simulink model "demoDINA_PCSSP"  (Simulink 8.0)
settings: Solver=ode1  SolverMode=SingleTasking  StartTime=0.0  StopTime=100.1  FixedStep=SimStep  RelTol=1e-3
InitFcn:
  | init_param_PCS6;
values from neighbouring files (symbols this model uses):
  n_gaps = 6    [init_param_PCS6.m]
  ncam = 100    [init_param_PCS6.m]
  npf = 15    [init_param_PCS6.m]
  SimStep = 2e-3    (= 0.002)    [init_param_PCS6.m]
  Time_stop = 1530    [init_param_PCS6.m]
undefined symbols (not defined in the file or in its folder): c_eob, dt_end_sim, dtpl_term_l, elong_ref, g1_ref, g1_ref_term, g2_ref, g2_ref_term, g3_ref, g3_ref_term, g4_ref, g4_ref_term, g5_ref, g5_ref_term, g6_ref, g6_ref_term, Ics1_eob, Ip_0, Ip_div, k_gaplim, n_mc, Ratemc_low, Ratemc_up, ref_ramp, scr_data, scr_PF, t_eob2, t_tran2D, Tfmc, Vmc_low, Vmc_up, VS_low, VS_up
libraries: simulink x5
settings Model: Creator=invite  LastModifiedBy=medveds  ExtModeAutoUpdateStatusClock=off  TunableVars=K,num  TunableVarsStorageClass=Auto,Auto  TunableVarsTypeQualifier=,  BufferReuse=off
settings DataIOCC: SignalLoggingSaveFormat=ModelDataLogs
settings OptimizationCC: BlockReduction=off  BooleanDataType=off  ConditionallyExecuteInputs=off  OptimizeBlockIOStorage=off  BufferReuse=off  ExpressionFolding=off  LocalBlockOutputs=off  InitFltsAndDblsToZero=on  AccelVerboseBuild=on
settings DebuggingCC: FcnCallInpInsideContextMsg=UseLocalSettings  SFcnCompatibilityMsg=warning  StrictBusMsg=Warning
settings SFSimCC: SimParseCustomCode=off  SimBuildMode=sf_make
settings CodeAppCC: CustomSymbolStrType=$N$R$M_T
settings GRTTargetCC: CombineOutputUpdateFcns=off  GRTInterface=on

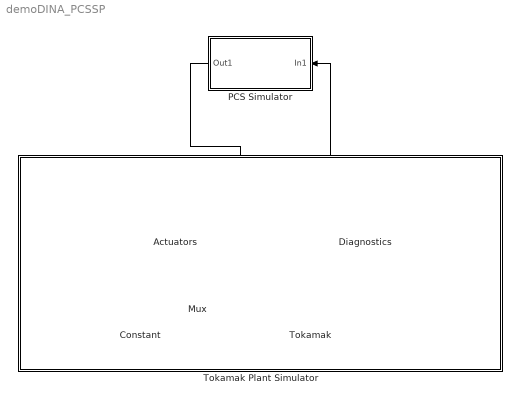
== system demoDINA_PCSSP ==
  Actuators : Subsystem
  Constant : Constant  Value=5  SampleTime=-1
  Diagnostics : Subsystem
  Mux : Mux  Inputs=2
  PCS Simulator : Subsystem
  Tokamak : S-Function  FunctionName=simimasdialogPCSSP  EnableBusSupport=off
  Tokamak Plant Simulator : Subsystem
      mask Display: disp(' ')
  wires:
  Mux/1 -> Tokamak/1
  Constant/1 -> Mux/2
  PCS Simulator/1(Out1) -> Actuators/1(In1)
  Actuators/1(Out1) -> Mux/1
  Tokamak/1 -> Diagnostics/1(In1)
  Diagnostics/1(Out1) -> PCS Simulator/1(In1)

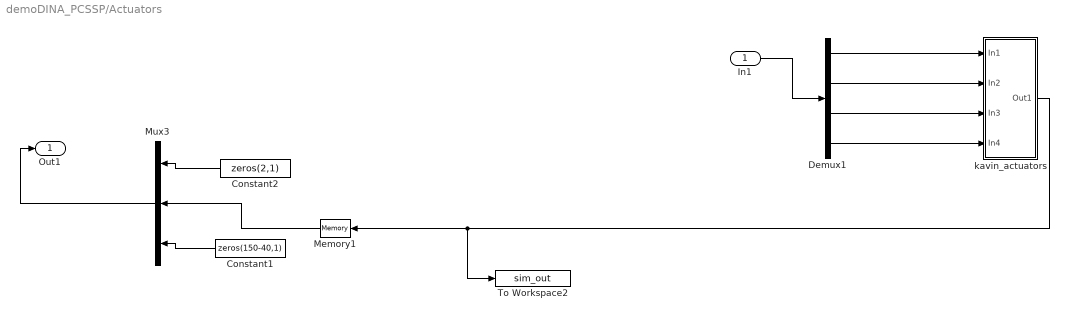
== system demoDINA_PCSSP/Actuators ==
  In1 : Inport
  Constant1 : Constant  Value=zeros(150-40,1)
  Constant2 : Constant  Value=zeros(2,1)
  Demux1 : Demux  Outputs=[n_mc 1 n_mc 12]
  Memory1 : Memory
  Mux3 : Mux  Inputs=3
  To Workspace2 : ToWorkspace  VariableName=sim_out
  kavin_actuators : Subsystem
  Out1 : Outport
  wires:
  In1/1 -> Demux1/1
  Mux3/1 -> Out1/1
  kavin_actuators/1(Out1) -> To Workspace2/1, Memory1/1
  Demux1/1 -> kavin_actuators/1(In1)
  Demux1/2 -> kavin_actuators/2(In2)
  Demux1/3 -> kavin_actuators/3(In3)
  Demux1/4 -> kavin_actuators/4(In4)
  Constant1/1 -> Mux3/3
  Memory1/1 -> Mux3/2
  Constant2/1 -> Mux3/1

== system demoDINA_PCSSP/Diagnostics ==
  In1 : Inport
  Out1 : Outport
  wires:
  In1/1 -> Out1/1

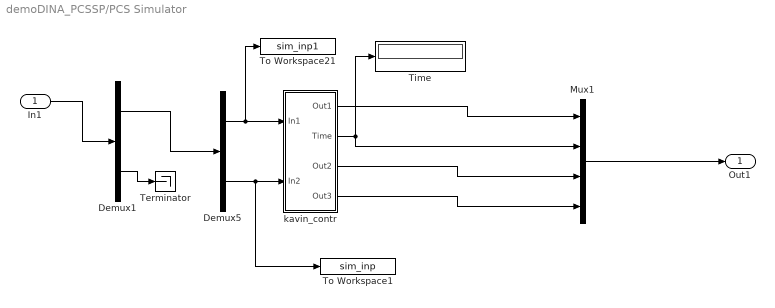
== system demoDINA_PCSSP/PCS Simulator ==
  In1 : Inport
  Demux1 : Demux  Outputs=[138 12]
  Demux5 : Demux  Outputs=[15 123]
  Mux1 : Mux
  Terminator : Terminator
  Time : Display
  To Workspace1 : ToWorkspace  VariableName=sim_inp
  To Workspace21 : ToWorkspace  VariableName=sim_inp1
  kavin_contr : Subsystem
  Out1 : Outport
  wires:
  Demux5/1 -> kavin_contr/1(In1), To Workspace21/1
  Demux5/2 -> kavin_contr/2(In2), To Workspace1/1
  Demux1/1 -> Demux5/1
  In1/1 -> Demux1/1
  Demux1/2 -> Terminator/1
  kavin_contr/2(Time) -> Mux1/2, Time/1
  kavin_contr/1(Out1) -> Mux1/1
  kavin_contr/3(Out2) -> Mux1/3
  kavin_contr/4(Out3) -> Mux1/4
  Mux1/1 -> Out1/1

== system demoDINA_PCSSP/Tokamak Plant Simulator ==

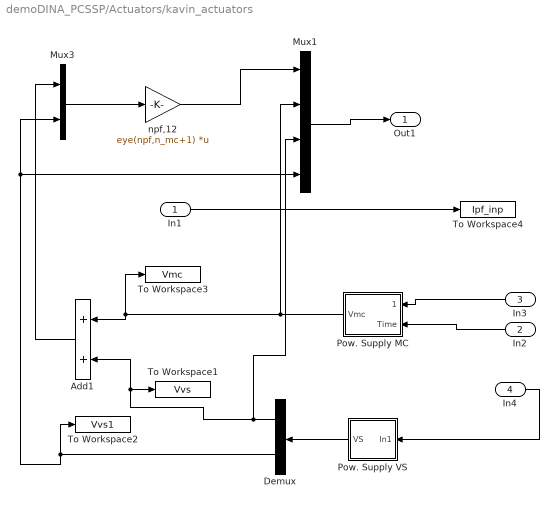
== system demoDINA_PCSSP/Actuators/kavin_actuators ==
  In1 : Inport
  In2 : Inport  Port=2
  In3 : Inport  Port=3
  In4 : Inport  Port=4
  Add1 : Sum
  Demux : Demux  Outputs=[n_mc 1]
  Mux1 : Mux
  Mux3 : Mux  Inputs=2
  "Pow. Supply MC " : Subsystem
  Pow. Supply VS : Subsystem
  To Workspace1 : ToWorkspace  VariableName=Vvs
  To Workspace2 : ToWorkspace  VariableName=Vvs1
  To Workspace3 : ToWorkspace  VariableName=Vmc
  To Workspace4 : ToWorkspace  VariableName=Ipf_inp
  npf,12 : Gain  Gain=eye(npf,n_mc+1)  Multiplication=Matrix(K*u)
  Out1 : Outport
  wires:
  Add1/1 -> Mux3/1
  Mux3/1 -> npf,12/1
  Demux/2 -> Mux1/4, Mux3/2, To Workspace2/1
  Demux/1 -> Mux1/3, To Workspace1/1, Add1/2
  In4/1 -> Pow. Supply VS/1(In1)
  Pow. Supply VS/1(VS) -> Demux/1
  In3/1 -> "Pow. Supply MC "/1(Vcontr)
  In2/1 -> "Pow. Supply MC "/2(Time)
  In1/1 -> To Workspace4/1
  npf,12/1 -> Mux1/1
  "Pow. Supply MC "/1(Vmc) -> Add1/1, To Workspace3/1, Mux1/2
  Mux1/1 -> Out1/1

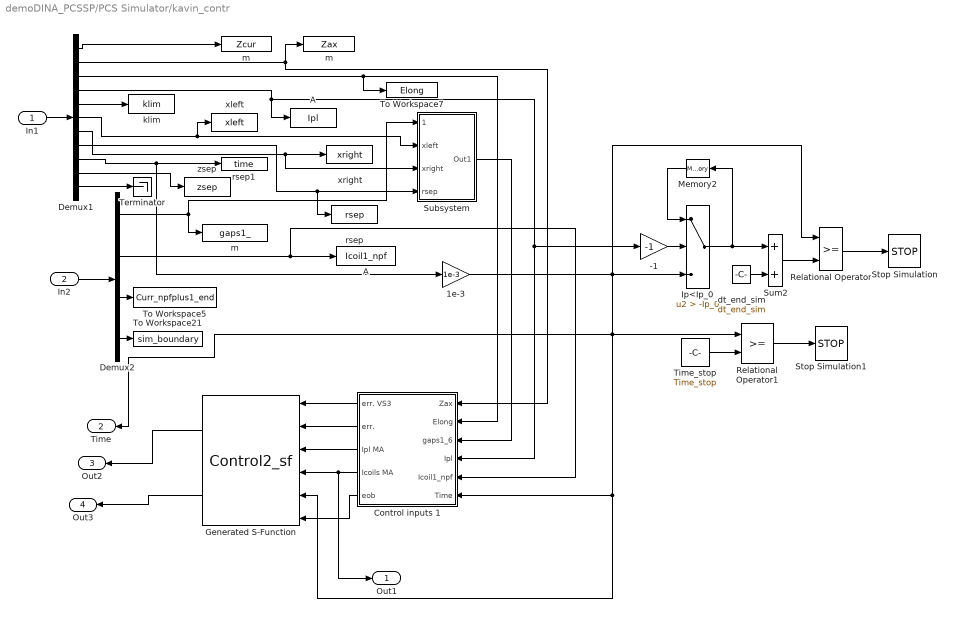
== system demoDINA_PCSSP/PCS Simulator/kavin_contr ==
  In1 : Inport
  In2 : Inport  Port=2
  -1 : Gain  Gain=-1
  1e-3 : Gain  Gain=1e-3
  A : ToWorkspace  VariableName=Ipl
  "A  " : ToWorkspace  VariableName=Icoil1_npf
  Control inputs 1 : Subsystem
  Demux1 : Demux  Outputs=[1 1 1 1 1 1 1 1 1 1 5 ]
  Demux2 : Demux  Outputs=[n_gaps npf ncam 2]
  Generated S-Function : S-Function  FunctionName=Control2_sf  SFunctionModules=""  EnableBusSupport=off  mask{rtw_sf_name=Control2_sf, showVar=off}
      mask prompts: rtw_sf_name "Simulink:masks:GenSFuncName_MP"; showVar "Simulink:masks:GenSFuncShowModuleList_MP"
      mask help: Simulink:masks:GenSFuncDesc_MD
      mask init:
      | displist = '';
      | if ~strcmp(get_param(gcb, 'FunctionName'), rtw_sf_name);
      |   set_param(gcb, 'FunctionName', rtw_sf_name);
      | end
      | % Check if we are generating code
      | rtw_mode = false;
      | if strcmpi(get_param(bdroot(gcb),'SimulationStatus'),'Initializing')
      | 	rtw_mode = strcmpi(get_param(bdroot(gcb),'BuildingRTWCode'),'on') && ...
      | 		~strcmpi(get_param(bdroot(gcb),'TargetStyle'),'SimulationTarget');
      | end
      | if showVar || rtw_mode
      | 	if exist('rtwsfunc') == 2 | exist('rtwsfunc') == 6
      | 		tmplist = rtwsfunc(rtw_sf_name,gcb);
      | 		tmplist = DAStudio.message('Simulink:masks:GenSFuncListOfModules_IC', tmplist);
      | 	elseif showVar
      | 		tmplist1 = DAStudio.message('Simulink:masks:GenSFuncListOfModules_IC', '');
      |         tmplist2 = DAStudio.message('Simulink:masks:GenSFuncNotLicensed_IC');
      |         tmplist = [tmplist1 tmplist2];
      |  	end
      | end
      | if showVar
      |   displist = tmplist;
      | end
      settings: CopyFcn=|
      | if ~strcmp(get_param(gcb,'Linkstatus'),'none') && ...
      | ~strcmp(get_param(gcb,'Linkstatus'),'implicit')
      |   set_param(gcb,'LinkStatus','none');
      | end
      mask Help: eval('feval(''rtwprivate'',''rtwhelpview'',''rtw_sfcn_block'')');
      mask Display:
      | port_label('input',1,'err. VS3');
      | port_label('input',2,'err.');
      | port_label('input',3,'Ipl MA');
      | port_label('input',4,'Icoils MA');
      | port_label('input',5,'Time');
      | port_label('input',6,'eob');
      | port_label('output',1,'Vmc control');
      | port_label('output',2,'Vvs control');
  "Ip<Ip_0 " : Switch  Criteria=u2 > Threshold  Threshold=-Ip_0
  Memory2 : Memory
  Relational Operator : RelationalOperator  OutDataTypeStr=boolean
  Relational Operator1 : RelationalOperator  OutDataTypeStr=boolean
  Stop Simulation : Stop
  Stop Simulation1 : Stop
  Subsystem : Subsystem
  Sum2 : Sum
  Terminator : Terminator
  Time_stop : Constant  Value=Time_stop
  To Workspace21 : ToWorkspace  VariableName=sim_boundary
      settings: Decimation=DecimShape
  To Workspace5 : ToWorkspace  VariableName=Curr_npfplus1_end
  To Workspace7 : ToWorkspace  VariableName=Elong
  dt_end_sim : Constant  Value=dt_end_sim
  klim : ToWorkspace  VariableName=klim
  m : ToWorkspace  VariableName=gaps1_
  "m  " : ToWorkspace  VariableName=Zax
  "m   " : ToWorkspace  VariableName=Zcur
  rsep : ToWorkspace  VariableName=rsep
  rsep1 : ToWorkspace  VariableName=time
  xleft : ToWorkspace  VariableName=xleft
  xright : ToWorkspace  VariableName=xright
  zsep : ToWorkspace  VariableName=zsep
  Out1 : Outport
  Time : Outport  Port=2
  Out2 : Outport  Port=3
  Out3 : Outport  Port=4
  wires:
  Demux1/2 -> "m  "/1, Control inputs 1/1(Zax)
  Demux1/1 -> "m   "/1
  Demux1/3 -> To Workspace7/1, Control inputs 1/2(Elong)
  Demux2/4 -> To Workspace21/1
  Demux1/4 -> A/1, Control inputs 1/4(Ipl), -1/1
  Demux2/3 -> To Workspace5/1
  Demux2/2 -> "A  "/1, Control inputs 1/5(Icoil1_npf)
  Control inputs 1/1(err. VS3) -> Generated S-Function/1
  Control inputs 1/2(err.) -> Generated S-Function/2
  Control inputs 1/3(Ipl MA) -> Generated S-Function/3
  Control inputs 1/4(Icoils MA) -> Out1/1, Generated S-Function/4
  In1/1 -> Demux1/1
  In2/1 -> Demux2/1
  Demux1/5 -> klim/1
  Demux1/6 -> xleft/1, Subsystem/2(xleft)
  Demux1/7 -> xright/1, Subsystem/3(xright)
  Demux1/8 -> rsep/1, Subsystem/4(rsep)
  Demux2/1 -> m/1, Subsystem/1(gaps1_6)
  Subsystem/1(Out1) -> Control inputs 1/3(gaps1_6)
  Demux1/11 -> Terminator/1
  Demux1/9 -> rsep1/1, 1e-3/1
  Demux1/10 -> zsep/1
  1e-3/1 -> "Ip<Ip_0 "/3, Relational Operator/1, Time/1, Generated S-Function/5, Control inputs 1/6(Time), Relational Operator1/1
  Relational Operator/1 -> Stop Simulation/1
  -1/1 -> "Ip<Ip_0 "/2
  "Ip<Ip_0 "/1 -> Memory2/1, Sum2/1
  Memory2/1 -> "Ip<Ip_0 "/1
  Sum2/1 -> Relational Operator/2
  dt_end_sim/1 -> Sum2/2
  Relational Operator1/1 -> Stop Simulation1/1
  Time_stop/1 -> Relational Operator1/2
  Control inputs 1/5(eob) -> Generated S-Function/6
  Generated S-Function/1 -> Out2/1
  Generated S-Function/2 -> Out3/1

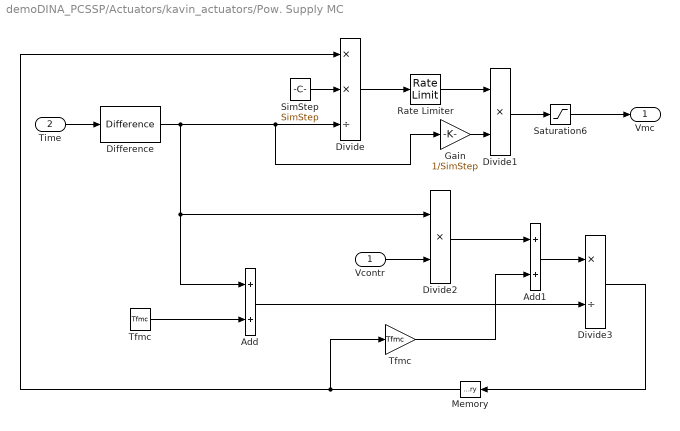
== system demoDINA_PCSSP/Actuators/kavin_actuators/Pow. Supply MC  ==
  Vcontr : Inport
  Time : Inport  Port=2
  Add : Sum
  Add1 : Sum
  Difference : simulink/Discrete/Difference  ICPrevInput=0.0  InputProcessing=Inherited  OutMin=[]  OutMax=[]  OutDataType=sfix(16)  OutScaling=2^-10  DoSatur=off
  Divide : Product  Inputs=**/
  Divide1 : Product  Inputs=**
  Divide2 : Product  Inputs=**
  Divide3 : Product  Inputs=*/
  Gain : Gain  Gain=1/SimStep
  Memory : Memory
  Rate Limiter : RateLimiter  RisingSlewLimit=Ratemc_up  FallingSlewLimit=Ratemc_low  SampleTimeMode=inherited
  Saturation6 : Saturate  UpperLimit=Vmc_up  LowerLimit=Vmc_low
  SimStep : Constant  Value=SimStep
  Tfmc : Constant  Value=Tfmc
  "Tfmc " : Gain  Gain=Tfmc
  Vmc : Outport
  wires:
  Saturation6/1 -> Vmc/1
  Time/1 -> Difference/1
  SimStep/1 -> Divide/2
  Difference/1 -> Divide/3, Gain/1, Divide2/1, Add/1
  Divide/1 -> Rate Limiter/1
  Rate Limiter/1 -> Divide1/1
  Divide1/1 -> Saturation6/1
  Gain/1 -> Divide1/2
  Tfmc/1 -> Add/2
  Divide2/1 -> Add1/1
  Memory/1 -> Divide/1, "Tfmc "/1
  Vcontr/1 -> Divide2/2
  "Tfmc "/1 -> Add1/2
  Add1/1 -> Divide3/1
  Divide3/1 -> Memory/1
  Add/1 -> Divide3/2

== system demoDINA_PCSSP/Actuators/kavin_actuators/Pow. Supply VS ==
  In1 : Inport
  Saturation VS : Saturate  UpperLimit=VS_up  LowerLimit=VS_low
  VS : Outport
  wires:
  In1/1 -> Saturation VS/1
  Saturation VS/1 -> VS/1

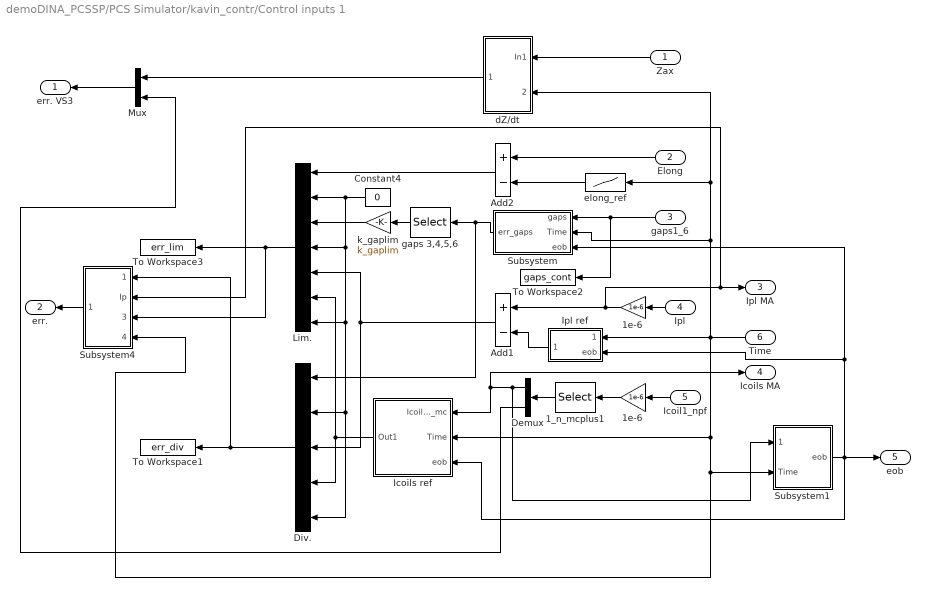
== system demoDINA_PCSSP/PCS Simulator/kavin_contr/Control inputs 1 ==
  Zax : Inport
  Elong : Inport  Port=2
  gaps1_6 : Inport  Port=3
  Ipl : Inport  Port=4
  Icoil1_npf : Inport  Port=5
  Time : Inport  Port=6
  1_n_mcplus1 : Selector  InputPortWidth=npf  IndexOptions=Index vector (dialog)  Indices=[1:n_mc+1]  OutputSizes=1
  1e-6 : Gain  Gain=1e-6
  "1e-6   " : Gain  Gain=1e-6
  Add1 : Sum  Inputs=+-
  Add2 : Sum  Inputs=+-
  Constant4 : Constant  Value=0  VectorParams1D=off
  Demux : Demux  Outputs=[n_mc 1]
  "Div. " : Mux  Inputs=5
  Icoils ref : Subsystem
  Ipl ref : Subsystem
  "Lim. " : Mux  Inputs=7
  Mux : Mux  Inputs=2
  Subsystem : Subsystem
  Subsystem1 : Subsystem
  Subsystem4 : Subsystem
  To Workspace1 : ToWorkspace  VariableName=err_div
  To Workspace2 : ToWorkspace  VariableName=gaps_cont
  To Workspace3 : ToWorkspace  VariableName=err_lim
  dZ/dt : Subsystem
  elong_ref : Lookup  InputValues=elong_ref(:,1)  Table=elong_ref(:,2)
  gaps 3,4,5,6 : Selector  InputPortWidth=6  IndexOptions=Index vector (dialog)  Indices=[3:6]  OutputSizes=1
  k_gaplim : Gain  Gain=k_gaplim
  err. VS3 : Outport
  err. : Outport  Port=2
  Ipl MA : Outport  Port=3
  Icoils MA : Outport  Port=4
  eob : Outport  Port=5
  wires:
  Zax/1 -> dZ/dt/1(In1)
  gaps1_6/1 -> To Workspace2/1, Subsystem/1(gaps)
  Ipl/1 -> 1e-6/1
  Icoil1_npf/1 -> "1e-6   "/1
  "1e-6   "/1 -> 1_n_mcplus1/1
  1_n_mcplus1/1 -> Demux/1
  Elong/1 -> Add2/1
  Ipl ref/1(Out1) -> Add1/2
  1e-6/1 -> Add1/1, Ipl MA/1, Subsystem4/2(Ip)
  Demux/1 -> Subsystem1/1(Icoils,MA), Icoils MA/1, Icoils ref/1(Icoil_n_mc)
  Add2/1 -> "Lim. "/1
  Constant4/1 -> "Lim. "/2, "Lim. "/4, "Lim. "/7, "Div. "/2, "Div. "/5
  gaps 3,4,5,6/1 -> k_gaplim/1
  Add1/1 -> "Lim. "/5, "Div. "/3
  Icoils ref/1(Out1) -> "Div. "/4, "Lim. "/6
  Subsystem/1(err_gaps) -> gaps 3,4,5,6/1, "Div. "/1
  Demux/2 -> Mux/2
  Mux/1 -> err. VS3/1
  "Div. "/1 -> To Workspace1/1, Subsystem4/1(err. div.)
  "Lim. "/1 -> Subsystem4/3(err. lim.), To Workspace3/1
  Subsystem4/1(Out1) -> err./1
  elong_ref/1 -> Add2/2
  dZ/dt/1(Out1) -> Mux/1
  k_gaplim/1 -> "Lim. "/3
  Time/1 -> elong_ref/1, dZ/dt/2(Time), Subsystem/2(Time), Icoils ref/2(Time), Subsystem4/4(Time), Subsystem1/2(Time), Ipl ref/1(Time)
  Subsystem1/1(eob) -> Icoils ref/3(eob), Subsystem/3(eob), Ipl ref/2(eob), eob/1

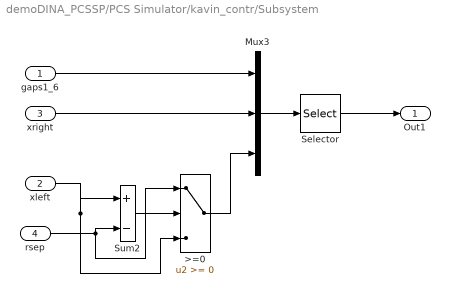
== system demoDINA_PCSSP/PCS Simulator/kavin_contr/Subsystem ==
  gaps1_6 : Inport
  xleft : Inport  Port=2
  xright : Inport  Port=3
  rsep : Inport  Port=4
  >=0 : Switch
  Mux3 : Mux  Inputs=3
  Selector : Selector  InputPortWidth=8  IndexOptions=Index vector (dialog)  Indices=[1 2 7 4 5 8]  OutputSizes=1
  Sum2 : Sum  Inputs=|+-
  Out1 : Outport
  wires:
  gaps1_6/1 -> Mux3/1
  rsep/1 -> Sum2/2, >=0/1
  Sum2/1 -> >=0/2
  xleft/1 -> Sum2/1, >=0/3
  >=0/1 -> Mux3/3
  xright/1 -> Mux3/2
  Mux3/1 -> Selector/1
  Selector/1 -> Out1/1

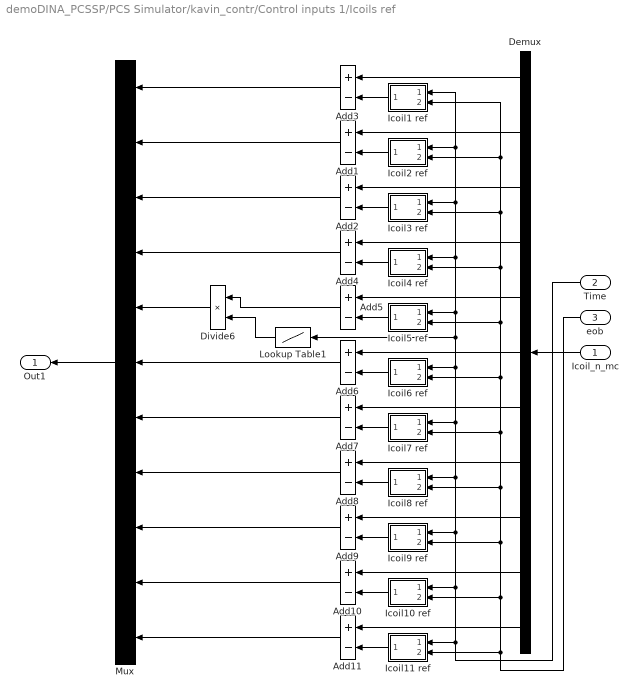
== system demoDINA_PCSSP/PCS Simulator/kavin_contr/Control inputs 1/Icoils ref ==
  Icoil_n_mc : Inport
  Time : Inport  Port=2
  eob : Inport  Port=3
  Add{1..11} (11 alike) : Sum  Inputs=+-
  Demux : Demux  Outputs=n_mc
  Divide6 : Product  Inputs=**
  Icoil1 ref : Subsystem
  Icoil10 ref : Subsystem
  Icoil11 ref : Subsystem
  Icoil2 ref : Subsystem
  Icoil3 ref : Subsystem
  Icoil4 ref : Subsystem
  Icoil5 ref : Subsystem
  Icoil6 ref : Subsystem
  Icoil7 ref : Subsystem
  Icoil8 ref : Subsystem
  Icoil9 ref : Subsystem
  Lookup Table1 : Lookup  InputValues=[0 t_tran2D t_tran2D+ref_ramp 1e6]  Table=[0 0 1 1]
  Mux : Mux  Inputs=n_mc
  Out1 : Outport
  wires:
  Icoil_n_mc/1 -> Demux/1
  Demux/1 -> Add3/1
  Time/1 -> Icoil11 ref/1(Time), Icoil10 ref/1(Time), Icoil9 ref/1(Time), Icoil8 ref/1(Time), Icoil7 ref/1(Time), Icoil6 ref/1(Time), Icoil4 ref/1(Time), Icoil3 ref/1(Time), Icoil2 ref/1(Time), Icoil1 ref/1(Time), Icoil5 ref/1(Time), Lookup Table1/1
  Icoil2 ref/1(Out1) -> Add1/2
  Demux/2 -> Add1/1
  Demux/3 -> Add2/1
  Icoil3 ref/1(Out1) -> Add2/2
  Icoil4 ref/1(Out1) -> Add4/2
  Demux/4 -> Add4/1
  Icoil5 ref/1(Out1) -> Add5/2
  Demux/5 -> Add5/1
  Icoil6 ref/1(Out1) -> Add6/2
  Demux/6 -> Add6/1
  Icoil7 ref/1(Out1) -> Add7/2
  Demux/7 -> Add7/1
  Icoil8 ref/1(Out1) -> Add8/2
  Demux/8 -> Add8/1
  Icoil9 ref/1(Out1) -> Add9/2
  Demux/9 -> Add9/1
  Icoil10 ref/1(Out1) -> Add10/2
  Demux/10 -> Add10/1
  Icoil11 ref/1(Out1) -> Add11/2
  Demux/11 -> Add11/1
  Add3/1 -> Mux/1
  Add1/1 -> Mux/2
  Add2/1 -> Mux/3
  Add4/1 -> Mux/4
  Add6/1 -> Mux/6
  Add7/1 -> Mux/7
  Add8/1 -> Mux/8
  Add9/1 -> Mux/9
  Add10/1 -> Mux/10
  Add11/1 -> Mux/11
  eob/1 -> Icoil11 ref/2(eob), Icoil10 ref/2(eob), Icoil9 ref/2(eob), Icoil8 ref/2(eob), Icoil7 ref/2(eob), Icoil6 ref/2(eob), Icoil4 ref/2(eob), Icoil3 ref/2(eob), Icoil2 ref/2(eob), Icoil1 ref/2(eob), Icoil5 ref/2(eob)
  Mux/1 -> Out1/1
  Add5/1 -> Divide6/1
  Lookup Table1/1 -> Divide6/2
  Divide6/1 -> Mux/5
  Icoil1 ref/1(Out1) -> Add3/2

== system demoDINA_PCSSP/PCS Simulator/kavin_contr/Control inputs 1/Ipl ref ==
  Time : Inport
  eob : Inport  Port=2
  Divide6 : Product  Inputs=**
  Ipl_ref : Lookup  InputValues=scr_data(:,1)  Table=scr_data(:,2)
  Memory1 : Memory
  c_eob : Switch  Criteria=u2 > Threshold  Threshold=c_eob
  Out1 : Outport
  wires:
  c_eob/1 -> Divide6/1, Memory1/1
  Divide6/1 -> Out1/1
  Time/1 -> Ipl_ref/1
  eob/1 -> Divide6/2, c_eob/2
  Ipl_ref/1 -> c_eob/1
  Memory1/1 -> c_eob/3

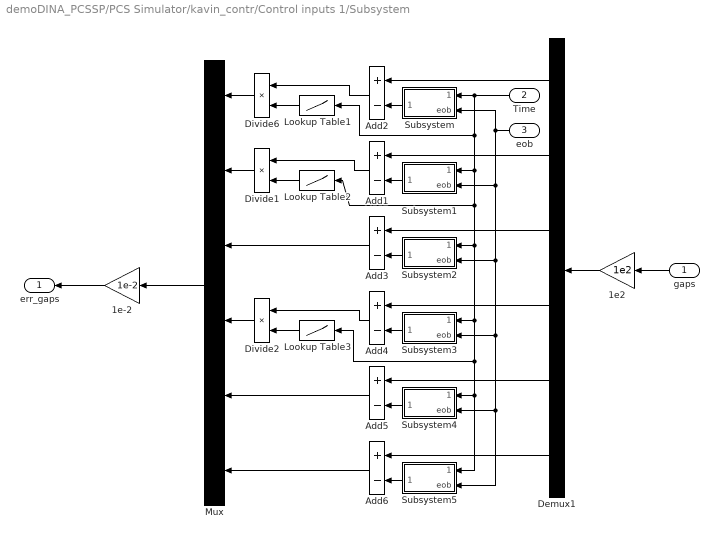
== system demoDINA_PCSSP/PCS Simulator/kavin_contr/Control inputs 1/Subsystem ==
  gaps : Inport
  Time : Inport  Port=2
  eob : Inport  Port=3
  1e-2 : Gain  Gain=1e-2
  1e2 : Gain  Gain=1e2
  Add{1..6} (6 alike) : Sum  Inputs=+-
  Demux1 : Demux  Outputs=6
  Divide1 : Product  Inputs=**
  Divide2 : Product  Inputs=**
  Divide6 : Product  Inputs=**
  Lookup Table1 : Lookup  InputValues=[0 t_tran2D t_tran2D+ref_ramp 1e6]  Table=[0 0 1 1]
  Lookup Table2 : Lookup  InputValues=[0 t_tran2D t_tran2D+ref_ramp 1e6]  Table=[0 0 1 1]
  Lookup Table3 : Lookup  InputValues=[0 t_tran2D t_tran2D+ref_ramp 1e6]  Table=[0 0 1 1]
  Mux : Mux  Inputs=6
  Subsystem : Subsystem
  Subsystem1 : Subsystem
  Subsystem2 : Subsystem
  Subsystem3 : Subsystem
  Subsystem4 : Subsystem
  Subsystem5 : Subsystem
  err_gaps : Outport
  wires:
  gaps/1 -> 1e2/1
  Time/1 -> Subsystem1/1(Time), Subsystem2/1(Time), Subsystem3/1(Time), Subsystem5/1(Time), Subsystem4/1(Time), Lookup Table3/1, Lookup Table2/1, Lookup Table1/1, Subsystem/1(Time)
  Demux1/1 -> Add2/1
  Demux1/2 -> Add1/1
  Subsystem1/1(Out1) -> Add1/2
  Subsystem2/1(Out1) -> Add3/2
  Demux1/3 -> Add3/1
  Demux1/4 -> Add4/1
  Subsystem3/1(Out1) -> Add4/2
  Demux1/5 -> Add5/1
  Subsystem4/1(Out1) -> Add5/2
  Demux1/6 -> Add6/1
  Add3/1 -> Mux/3
  Add5/1 -> Mux/5
  Add6/1 -> Mux/6
  Mux/1 -> 1e-2/1
  1e2/1 -> Demux1/1
  Divide6/1 -> Mux/1
  Add2/1 -> Divide6/1
  Lookup Table1/1 -> Divide6/2
  Divide1/1 -> Mux/2
  Add1/1 -> Divide1/1
  Lookup Table2/1 -> Divide1/2
  Divide2/1 -> Mux/4
  Add4/1 -> Divide2/1
  Lookup Table3/1 -> Divide2/2
  1e-2/1 -> err_gaps/1
  Subsystem/1(Out1) -> Add2/2
  eob/1 -> Subsystem/2(eob), Subsystem3/2(eob), Subsystem5/2(eob), Subsystem4/2(eob), Subsystem2/2(eob), Subsystem1/2(eob)
  Subsystem5/1(Out1) -> Add6/2

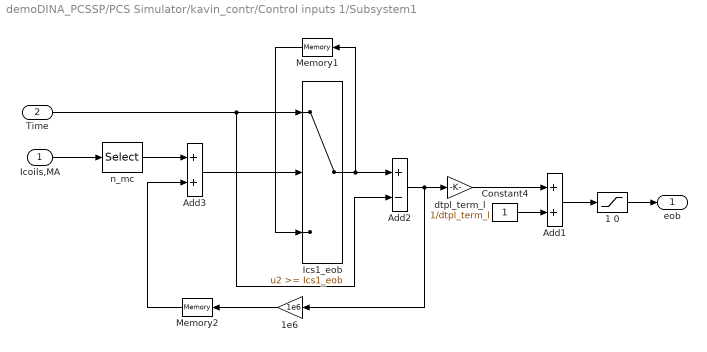
== system demoDINA_PCSSP/PCS Simulator/kavin_contr/Control inputs 1/Subsystem1 ==
  Icoils,MA : Inport
  Time : Inport  Port=2
  1 0 : Saturate  UpperLimit=1  LowerLimit=0
  1e6 : Gain  Gain=1e6
  Add1 : Sum
  Add2 : Sum  Inputs=+-
  Add3 : Sum
  Constant4 : Constant  VectorParams1D=off
  Ics1_eob : Switch  Threshold=Ics1_eob
  Memory1 : Memory
  Memory2 : Memory
  dtpl_term_l : Gain  Gain=1/dtpl_term_l
  n_mc : Selector  InputPortWidth=n_mc  IndexOptions=Index vector (dialog)  Indices=3  OutputSizes=1
  eob : Outport
  wires:
  Time/1 -> Add2/2, Ics1_eob/1
  Ics1_eob/1 -> Add2/1, Memory1/1
  Add2/1 -> 1e6/1, dtpl_term_l/1
  dtpl_term_l/1 -> Add1/1
  Constant4/1 -> Add1/2
  Add1/1 -> 1 0/1
  1 0/1 -> eob/1
  Memory1/1 -> Ics1_eob/3
  n_mc/1 -> Add3/1
  Add3/1 -> Ics1_eob/2
  1e6/1 -> Memory2/1
  Icoils,MA/1 -> n_mc/1
  Memory2/1 -> Add3/2

== system demoDINA_PCSSP/PCS Simulator/kavin_contr/Control inputs 1/Subsystem4 ==
  err. div. : Inport
  Ip : Inport  Port=2
  err. lim. : Inport  Port=3
  Time : Inport  Port=4
  0.99 : Switch  Threshold=0.99
  Compare To Constant : simulink/Logic and Bit Operations/Compare To Constant  relop=>  const=Ip_div  OutDataTypeStr=uint8  ZeroCross=off
  Compare To Constant1 : simulink/Logic and Bit Operations/Compare To Constant  relop=>  const=t_eob2  OutDataTypeStr=uint8  ZeroCross=off
  Logical Operator1 : Logic  Operator=OR  AllPortsSameDT=off  OutDataTypeStr=float('double')
  Out1 : Outport
  wires:
  0.99/1 -> Out1/1
  err. div./1 -> 0.99/1
  err. lim./1 -> 0.99/3
  Compare To Constant/1 -> Logical Operator1/1
  Compare To Constant1/1 -> Logical Operator1/2
  Time/1 -> Compare To Constant1/1
  Ip/1 -> Compare To Constant/1
  Logical Operator1/1 -> 0.99/2

== system demoDINA_PCSSP/PCS Simulator/kavin_contr/Control inputs 1/dZ/dt ==
  In1 : Inport
  Time : Inport  Port=2
  Difference : simulink/Discrete/Difference  ICPrevInput=0.0  InputProcessing=Inherited  OutMin=[]  OutMax=[]  OutDataType=sfix(16)  OutScaling=2^-10  DoSatur=off
  Difference1 : simulink/Discrete/Difference  ICPrevInput=0  InputProcessing=Inherited  OutMin=[]  OutMax=[]  OutDataType=sfix(16)  OutScaling=2^-10  DoSatur=off
  Divide : Product  Inputs=*/
  Out1 : Outport
  wires:
  In1/1 -> Difference/1
  Time/1 -> Difference1/1
  Difference/1 -> Divide/1
  Difference1/1 -> Divide/2
  Divide/1 -> Out1/1

== system demoDINA_PCSSP/PCS Simulator/kavin_contr/Control inputs 1/Icoils ref/Icoil1 ref ==
  Time : Inport
  eob : Inport  Port=2
  Divide1 : Product  Inputs=**
  Icoil1_ref : Lookup  InputValues=scr_PF(:,1)  Table=scr_PF(:,2)
  Memory2 : Memory
  c_eob : Switch  Criteria=u2 > Threshold  Threshold=c_eob
  Out1 : Outport
  wires:
  c_eob/1 -> Divide1/1, Memory2/1
  Divide1/1 -> Out1/1
  Time/1 -> Icoil1_ref/1
  eob/1 -> Divide1/2, c_eob/2
  Icoil1_ref/1 -> c_eob/1
  Memory2/1 -> c_eob/3

== system demoDINA_PCSSP/PCS Simulator/kavin_contr/Control inputs 1/Icoils ref/Icoil10 ref ==
  Time : Inport
  eob : Inport  Port=2
  Divide1 : Product  Inputs=**
  Icoil10_ref : Lookup  InputValues=scr_PF(:,1)  Table=scr_PF(:,11)
  Memory2 : Memory
  c_eob : Switch  Criteria=u2 > Threshold  Threshold=c_eob
  Out1 : Outport
  wires:
  c_eob/1 -> Divide1/1, Memory2/1
  Divide1/1 -> Out1/1
  Time/1 -> Icoil10_ref/1
  eob/1 -> Divide1/2, c_eob/2
  Icoil10_ref/1 -> c_eob/1
  Memory2/1 -> c_eob/3

== system demoDINA_PCSSP/PCS Simulator/kavin_contr/Control inputs 1/Icoils ref/Icoil11 ref ==
  Time : Inport
  eob : Inport  Port=2
  Divide1 : Product  Inputs=**
  Icoil11_ref : Lookup  InputValues=scr_PF(:,1)  Table=scr_PF(:,12)
  Memory2 : Memory
  c_eob : Switch  Criteria=u2 > Threshold  Threshold=c_eob
  Out1 : Outport
  wires:
  c_eob/1 -> Divide1/1, Memory2/1
  Divide1/1 -> Out1/1
  Time/1 -> Icoil11_ref/1
  eob/1 -> Divide1/2, c_eob/2
  Icoil11_ref/1 -> c_eob/1
  Memory2/1 -> c_eob/3

== system demoDINA_PCSSP/PCS Simulator/kavin_contr/Control inputs 1/Icoils ref/Icoil2 ref ==
  Time : Inport
  eob : Inport  Port=2
  Divide1 : Product  Inputs=**
  Icoil2_ref : Lookup  InputValues=scr_PF(:,1)  Table=scr_PF(:,3)
  Memory2 : Memory
  c_eob : Switch  Criteria=u2 > Threshold  Threshold=c_eob
  Out1 : Outport
  wires:
  c_eob/1 -> Divide1/1, Memory2/1
  Divide1/1 -> Out1/1
  Time/1 -> Icoil2_ref/1
  eob/1 -> Divide1/2, c_eob/2
  Icoil2_ref/1 -> c_eob/1
  Memory2/1 -> c_eob/3

== system demoDINA_PCSSP/PCS Simulator/kavin_contr/Control inputs 1/Icoils ref/Icoil3 ref ==
  Time : Inport
  eob : Inport  Port=2
  Divide1 : Product  Inputs=**
  Icoil3_ref : Lookup  InputValues=scr_PF(:,1)  Table=scr_PF(:,4)
  Memory2 : Memory
  c_eob : Switch  Criteria=u2 > Threshold  Threshold=c_eob
  Out1 : Outport
  wires:
  c_eob/1 -> Divide1/1, Memory2/1
  Divide1/1 -> Out1/1
  Time/1 -> Icoil3_ref/1
  eob/1 -> Divide1/2, c_eob/2
  Icoil3_ref/1 -> c_eob/1
  Memory2/1 -> c_eob/3

== system demoDINA_PCSSP/PCS Simulator/kavin_contr/Control inputs 1/Icoils ref/Icoil4 ref ==
  Time : Inport
  eob : Inport  Port=2
  Divide1 : Product  Inputs=**
  Icoil4_ref : Lookup  InputValues=scr_PF(:,1)  Table=scr_PF(:,5)
  Memory2 : Memory
  c_eob : Switch  Criteria=u2 > Threshold  Threshold=c_eob
  Out1 : Outport
  wires:
  c_eob/1 -> Divide1/1, Memory2/1
  Divide1/1 -> Out1/1
  Time/1 -> Icoil4_ref/1
  eob/1 -> Divide1/2, c_eob/2
  Icoil4_ref/1 -> c_eob/1
  Memory2/1 -> c_eob/3

== system demoDINA_PCSSP/PCS Simulator/kavin_contr/Control inputs 1/Icoils ref/Icoil5 ref ==
  Time : Inport
  eob : Inport  Port=2
  Divide1 : Product  Inputs=**
  Icoil5_ref : Lookup  InputValues=scr_PF(:,1)  Table=scr_PF(:,6)
  Memory2 : Memory
  c_eob : Switch  Criteria=u2 > Threshold  Threshold=c_eob
  Out1 : Outport
  wires:
  c_eob/1 -> Divide1/1, Memory2/1
  Divide1/1 -> Out1/1
  Time/1 -> Icoil5_ref/1
  eob/1 -> Divide1/2, c_eob/2
  Icoil5_ref/1 -> c_eob/1
  Memory2/1 -> c_eob/3

== system demoDINA_PCSSP/PCS Simulator/kavin_contr/Control inputs 1/Icoils ref/Icoil6 ref ==
  Time : Inport
  eob : Inport  Port=2
  Divide1 : Product  Inputs=**
  Icoil6_ref : Lookup  InputValues=scr_PF(:,1)  Table=scr_PF(:,7)
  Memory2 : Memory
  c_eob : Switch  Criteria=u2 > Threshold  Threshold=c_eob
  Out1 : Outport
  wires:
  c_eob/1 -> Divide1/1, Memory2/1
  Divide1/1 -> Out1/1
  Time/1 -> Icoil6_ref/1
  eob/1 -> Divide1/2, c_eob/2
  Icoil6_ref/1 -> c_eob/1
  Memory2/1 -> c_eob/3

== system demoDINA_PCSSP/PCS Simulator/kavin_contr/Control inputs 1/Icoils ref/Icoil7 ref ==
  Time : Inport
  eob : Inport  Port=2
  Divide1 : Product  Inputs=**
  Icoil1_ref : Lookup  InputValues=scr_PF(:,1)  Table=scr_PF(:,8)
  Memory2 : Memory
  c_eob : Switch  Criteria=u2 > Threshold  Threshold=c_eob
  Out1 : Outport
  wires:
  c_eob/1 -> Divide1/1, Memory2/1
  Divide1/1 -> Out1/1
  Time/1 -> Icoil1_ref/1
  eob/1 -> Divide1/2, c_eob/2
  Icoil1_ref/1 -> c_eob/1
  Memory2/1 -> c_eob/3

== system demoDINA_PCSSP/PCS Simulator/kavin_contr/Control inputs 1/Icoils ref/Icoil8 ref ==
  Time : Inport
  eob : Inport  Port=2
  Divide1 : Product  Inputs=**
  Icoil8_ref : Lookup  InputValues=scr_PF(:,1)  Table=scr_PF(:,9)
  Memory2 : Memory
  c_eob : Switch  Criteria=u2 > Threshold  Threshold=c_eob
  Out1 : Outport
  wires:
  c_eob/1 -> Divide1/1, Memory2/1
  Divide1/1 -> Out1/1
  Time/1 -> Icoil8_ref/1
  eob/1 -> Divide1/2, c_eob/2
  Icoil8_ref/1 -> c_eob/1
  Memory2/1 -> c_eob/3

== system demoDINA_PCSSP/PCS Simulator/kavin_contr/Control inputs 1/Icoils ref/Icoil9 ref ==
  Time : Inport
  eob : Inport  Port=2
  Divide1 : Product  Inputs=**
  Icoil9_ref : Lookup  InputValues=scr_PF(:,1)  Table=scr_PF(:,10)
  Memory2 : Memory
  c_eob : Switch  Criteria=u2 > Threshold  Threshold=c_eob
  Out1 : Outport
  wires:
  c_eob/1 -> Divide1/1, Memory2/1
  Divide1/1 -> Out1/1
  Time/1 -> Icoil9_ref/1
  eob/1 -> Divide1/2, c_eob/2
  Icoil9_ref/1 -> c_eob/1
  Memory2/1 -> c_eob/3

== system demoDINA_PCSSP/PCS Simulator/kavin_contr/Control inputs 1/Subsystem/Subsystem ==
  Time : Inport
  eob : Inport  Port=2
  Add2 : Sum  Inputs=-+
  Memory1 : Memory
  c_eob : Switch  Criteria=u2 > Threshold  Threshold=c_eob
  "c_eob  " : Switch  Criteria=u2 > Threshold  Threshold=c_eob
  g1_ref : Lookup  InputValues=g1_ref(:,1)  Table=g1_ref(:,2)
  g1_ref_term : Lookup  InputValues=g1_ref_term(:,1)  Table=g1_ref_term(:,2)
  Out1 : Outport
  wires:
  eob/1 -> "c_eob  "/2, c_eob/2
  Time/1 -> Add2/2, "c_eob  "/1, g1_ref/1
  g1_ref/1 -> c_eob/1
  "c_eob  "/1 -> Add2/1, Memory1/1
  Memory1/1 -> "c_eob  "/3
  Add2/1 -> g1_ref_term/1
  g1_ref_term/1 -> c_eob/3
  c_eob/1 -> Out1/1

== system demoDINA_PCSSP/PCS Simulator/kavin_contr/Control inputs 1/Subsystem/Subsystem1 ==
  Time : Inport
  eob : Inport  Port=2
  Add2 : Sum  Inputs=-+
  Memory1 : Memory
  c_eob : Switch  Criteria=u2 > Threshold  Threshold=c_eob
  "c_eob " : Switch  Criteria=u2 > Threshold  Threshold=c_eob
  g2_ref : Lookup  InputValues=g2_ref(:,1)  Table=g2_ref(:,2)
  g2_ref_term : Lookup  InputValues=g2_ref_term(:,1)  Table=g2_ref_term(:,2)
  Out1 : Outport
  wires:
  eob/1 -> "c_eob "/2, c_eob/2
  Time/1 -> Add2/2, "c_eob "/1, g2_ref/1
  g2_ref/1 -> c_eob/1
  "c_eob "/1 -> Add2/1, Memory1/1
  Memory1/1 -> "c_eob "/3
  Add2/1 -> g2_ref_term/1
  g2_ref_term/1 -> c_eob/3
  c_eob/1 -> Out1/1

== system demoDINA_PCSSP/PCS Simulator/kavin_contr/Control inputs 1/Subsystem/Subsystem2 ==
  Time : Inport
  eob : Inport  Port=2
  Add2 : Sum  Inputs=-+
  Memory1 : Memory
  c_eob : Switch  Criteria=u2 > Threshold  Threshold=c_eob
  "c_eob " : Switch  Criteria=u2 > Threshold  Threshold=c_eob
  g3_ref : Lookup  InputValues=g3_ref(:,1)  Table=g3_ref(:,2)
  g3_ref_term : Lookup  InputValues=g3_ref_term(:,1)  Table=g3_ref_term(:,2)
  Out1 : Outport
  wires:
  eob/1 -> "c_eob "/2, c_eob/2
  Time/1 -> Add2/2, "c_eob "/1, g3_ref/1
  g3_ref/1 -> c_eob/1
  "c_eob "/1 -> Add2/1, Memory1/1
  Memory1/1 -> "c_eob "/3
  Add2/1 -> g3_ref_term/1
  g3_ref_term/1 -> c_eob/3
  c_eob/1 -> Out1/1

== system demoDINA_PCSSP/PCS Simulator/kavin_contr/Control inputs 1/Subsystem/Subsystem3 ==
  Time : Inport
  eob : Inport  Port=2
  Add2 : Sum  Inputs=-+
  Memory1 : Memory
  c_eob : Switch  Criteria=u2 > Threshold  Threshold=c_eob
  "c_eob  " : Switch  Criteria=u2 > Threshold  Threshold=c_eob
  g4_ref : Lookup  InputValues=g4_ref(:,1)  Table=g4_ref(:,2)
  g4_ref_term : Lookup  InputValues=g4_ref_term(:,1)  Table=g4_ref_term(:,2)
  Out1 : Outport
  wires:
  eob/1 -> "c_eob  "/2, c_eob/2
  Time/1 -> Add2/2, "c_eob  "/1, g4_ref/1
  g4_ref/1 -> c_eob/1
  "c_eob  "/1 -> Add2/1, Memory1/1
  Memory1/1 -> "c_eob  "/3
  Add2/1 -> g4_ref_term/1
  g4_ref_term/1 -> c_eob/3
  c_eob/1 -> Out1/1

== system demoDINA_PCSSP/PCS Simulator/kavin_contr/Control inputs 1/Subsystem/Subsystem4 ==
  Time : Inport
  eob : Inport  Port=2
  Add2 : Sum  Inputs=-+
  Memory1 : Memory
  c_eob : Switch  Criteria=u2 > Threshold  Threshold=c_eob
  "c_eob  " : Switch  Criteria=u2 > Threshold  Threshold=c_eob
  g5_ref : Lookup  InputValues=g5_ref(:,1)  Table=g5_ref(:,2)
  g5_ref_term : Lookup  InputValues=g5_ref_term(:,1)  Table=g5_ref_term(:,2)
  Out1 : Outport
  wires:
  eob/1 -> "c_eob  "/2, c_eob/2
  Time/1 -> Add2/2, "c_eob  "/1, g5_ref/1
  g5_ref/1 -> c_eob/1
  "c_eob  "/1 -> Add2/1, Memory1/1
  Memory1/1 -> "c_eob  "/3
  Add2/1 -> g5_ref_term/1
  g5_ref_term/1 -> c_eob/3
  c_eob/1 -> Out1/1

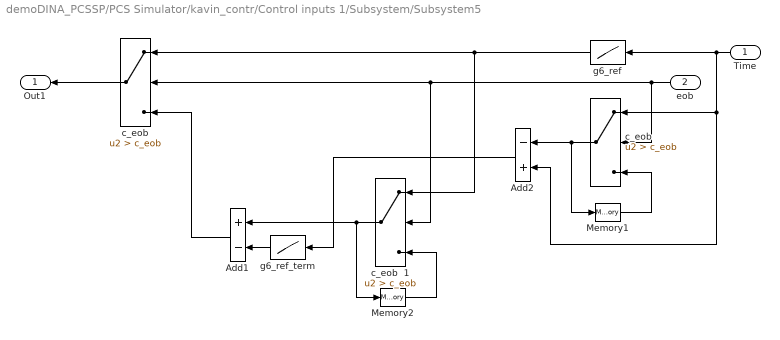
== system demoDINA_PCSSP/PCS Simulator/kavin_contr/Control inputs 1/Subsystem/Subsystem5 ==
  Time : Inport
  eob : Inport  Port=2
  Add1 : Sum  Inputs=+-
  Add2 : Sum  Inputs=-+
  Memory1 : Memory
  Memory2 : Memory
  c_eob : Switch  Criteria=u2 > Threshold  Threshold=c_eob
  "c_eob  " : Switch  Criteria=u2 > Threshold  Threshold=c_eob
  c_eob  1 : Switch  Criteria=u2 > Threshold  Threshold=c_eob
  g6_ref : Lookup  InputValues=g6_ref(:,1)  Table=g6_ref(:,2)
  g6_ref_term : Lookup  InputValues=g6_ref_term(:,1)  Table=g6_ref_term(:,2)
  Out1 : Outport
  wires:
  Time/1 -> Add2/2, "c_eob  "/1, g6_ref/1
  "c_eob  "/1 -> Add2/1, Memory1/1
  Memory1/1 -> "c_eob  "/3
  Add2/1 -> g6_ref_term/1
  c_eob/1 -> Out1/1
  eob/1 -> "c_eob  "/2, c_eob  1/2, c_eob/2
  g6_ref/1 -> c_eob  1/1, c_eob/1
  c_eob  1/1 -> Memory2/1, Add1/1
  Memory2/1 -> c_eob  1/3
  g6_ref_term/1 -> Add1/2
  Add1/1 -> c_eob/3
